simulink model "ControlsWithAutopilot_Properties"  (R2016a)
settings: Solver=ode45  StartTime=0.0  StopTime=10.0  RelTol=1e-3
undefined symbols (not defined in the file): ap, bias, DiscIntNeverNeededParam
libraries: simulink x3, discretizing x1
(part 1 of 3)
settings Model: Creator=mddavies  LastModifiedBy=Teme
settings DataIOCC: LimitDataPoints=on  SaveFormat=Array  SignalLoggingSaveFormat=ModelDataLogs
settings DebuggingCC: UnderspecifiedInitializationDetection=Classic  MergeDetectMultiDrivingBlocksExec=none  SolverPrmCheckMsg=warning  FcnCallInpInsideContextMsg=UseLocalSettings  StateNameClashWarn=warning
settings HardwareCC: ProdBitPerPointer=32  ProdLargestAtomicFloat=None  ProdIntDivRoundTo=Undefined  ProdEndianess=Unspecified  ProdWordSize=32  ProdHWDeviceType=32-bit Generic
settings ModelReferenceCC: PropagateSignalLabelsOutOfModel=off
settings GRTTargetCC: CombineOutputUpdateFcns=off  GRTInterface=on
settings ConfigComp: CovModelRefEnable=Off  CovSFcnEnable=off

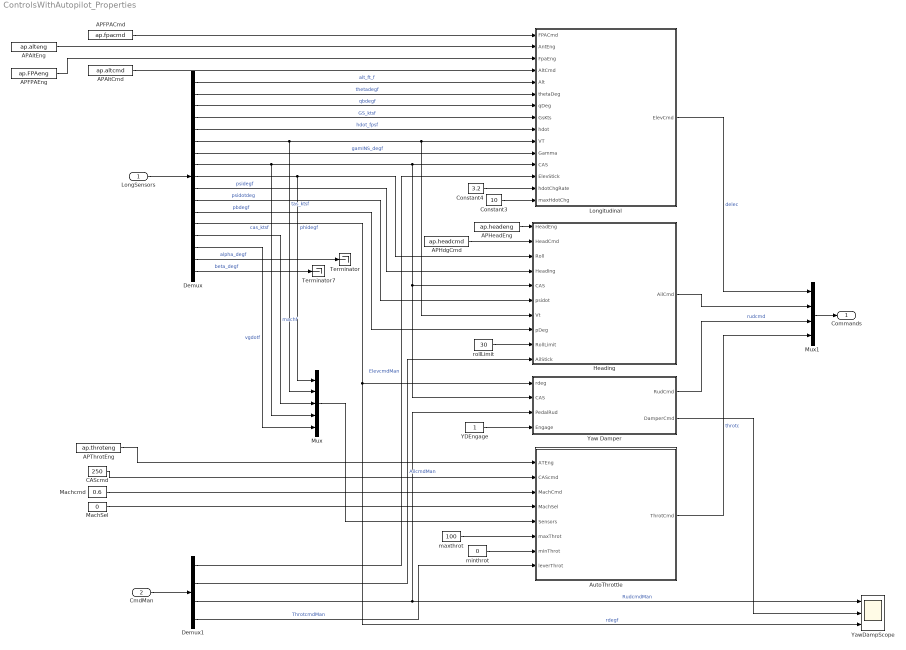
== system ControlsWithAutopilot_Properties ==
  LongSensors : Inport  RequirementInfo={} %GIDa_0ce9b168_5661_42b0_b4cb_7d3faaf2df72  PortDimensions=17
  CmdMan : Inport  RequirementInfo={} %GIDa_0ce9b168_5661_42b0_b4cb_7d3faaf2df72  Port=2  PortDimensions=9
  APAltCmd : Constant  RequirementInfo={} %GIDa_8396ea73_c2c1_410d_8e72_0a2c2e115229  Value=ap.altcmd
  APAltEng : Constant  RequirementInfo={} %GIDa_7acdc276_5904_4f5d_a4d8_b7eafc22dcba  Value=ap.alteng  OutDataTypeStr=boolean
  "APFPACmd " : Constant  RequirementInfo={} %GIDa_f2a9802e_c9ff_44b4_9c39_101c70e3085f  Value=ap.fpacmd
  APFPAEng : Constant  RequirementInfo={} %GIDa_b6347d6f_b14e_46b8_b79f_c4482e372009  Value=ap.FPAeng  OutDataTypeStr=boolean
  APHdgCmd : Constant  RequirementInfo={} %GIDa_ca348917_806b_4c73_b099_958ce531bbd5  Value=ap.headcmd
  APHeadEng : Constant  RequirementInfo={} %GIDa_019c8883_de5f_448b_a478_e0a40c975d97  Value=ap.headeng  OutDataTypeStr=boolean
  APThrotEng : Constant  RequirementInfo={} %GIDa_c34ca1b2_b760_48cb_8815_eaf096d766de  Value=ap.throteng  OutDataTypeStr=boolean
  AutoThrottle : Subsystem  RequirementInfo={'other' '..\..\tcm_requirements.docx' '@Simulink_requirement_item_20' 'true' 'Auto Throttle' '' } %GIDa_9e91f8aa_3697_4e86_a547_8b20eda6b794  TreatAsAtomicUnit=on
  CAScmd : Constant  RequirementInfo={} %GIDa_47d34f1f_8d24_42cb_857b_a6284aa9b10f  Value=250
  Constant3 : Constant  RequirementInfo={} %GIDa_6046f9e1_21da_4401_862c_288f604e8689  Value=10
  Constant4 : Constant  RequirementInfo={} %GIDa_dee93be0_a932_4ef0_a207_8f7329b01ca5  Value=3.2
  Demux : Demux  Outputs=17
  Demux1 : Demux
  Heading : Subsystem  TreatAsAtomicUnit=on
  Longitudinal : Subsystem  TreatAsAtomicUnit=on
  MachSel : Constant  RequirementInfo={} %GIDa_703eecf9_8ffd_4677_9df1_b11ad3ff81be  Value=0
  Machcmd : Constant  RequirementInfo={} %GIDa_a015b01e_abfd_4965_a258_bc3318cb77ef  Value=0.6
  Mux : Mux  Inputs=5
  Mux1 : Mux
  Terminator : Terminator
  Terminator7 : Terminator
      settings: RequirementInfo={} %GIDa_ea750fcf_3a35_4ca3_ba61_16c7ba83d83d
  YDEngage : Constant  RequirementInfo={} %GIDa_1b340559_9c71_403c_9901_bf0a93e2b9fd  SampleTime=-1
  Yaw Damper : Subsystem  RequirementInfo={'other' '..\..\tcm_requirements.docx' '@Simulink_requirement_item_19' 'true' 'Yaw Damper' '' } %GIDa_4d9fd165_a151_41ab_8542_450c342372eb  TreatAsAtomicUnit=on
  YawDampScope : Scope  NumInputPorts=3
      settings: RequirementInfo={} %GIDa_7592f6f2_c7e8_4acc_8768_b20cb3da46c8
  maxthrot : Constant  RequirementInfo={} %GIDa_230ab06c_3fb9_421e_bdda_8f032886ed67  Value=100  SampleTime=-1
  minthrot : Constant  RequirementInfo={} %GIDa_e24cf5cf_680d_403e_8bf4_a3705f2cf8ca  Value=0  SampleTime=-1
  rollLimit : Constant  RequirementInfo={} %GIDa_80188ac9_3eb7_4583_8db0_ebf7b7448de5  Value=30  SampleTime=-1
  Commands : Outport  RequirementInfo={} %GIDa_ba9bc9f0_2997_4cec_8a5a_2cb65716cddf
  wires:
  AutoThrottle/1(ThrotCmd) -> Mux1/4  "throtc"
  Longitudinal/1(ElevCmd) -> Mux1/1  "delec"
  Heading/1(AilCmd) -> Mux1/2
  CAScmd/1 -> AutoThrottle/2(CAScmd)
  APAltEng/1 -> Longitudinal/2(AntEng)
  Machcmd/1 -> AutoThrottle/3(MachCmd)
  MachSel/1 -> AutoThrottle/4(MachSel)
  APHeadEng/1 -> Heading/1(HeadEng)
  APFPAEng/1 -> Longitudinal/3(FpaEng)
  APThrotEng/1 -> AutoThrottle/1(ATEng)
  APHdgCmd/1 -> Heading/2(HeadCmd)
  "APFPACmd "/1 -> Longitudinal/1(FPACmd)
  APAltCmd/1 -> Longitudinal/4(AltCmd)
  maxthrot/1 -> AutoThrottle/6(maxThrot)
  Yaw Damper/2(DamperCmd) -> YawDampScope/2
  Yaw Damper/1(RudCmd) -> Mux1/3  "rudcmd"
  Constant3/1 -> Longitudinal/15(maxHdotChg)
  Constant4/1 -> Longitudinal/14(hdotChgRate)
  YDEngage/1 -> Yaw Damper/4(Engage)
  rollLimit/1 -> Heading/9(RollLimit)
  LongSensors/1 -> Demux/1
  Demux/1 -> Longitudinal/5(Alt)  "alt_ft_f"
  Demux/2 -> Longitudinal/6(thetaDeg)  "thetadegf"
  Demux/4 -> Longitudinal/8(GsKts)  "GS_ktsf"
  Demux/3 -> Longitudinal/7(qDeg)  "qbdegf"
  Demux/5 -> Longitudinal/9(hdot)  "hdot_fpsf"
  Demux/6 -> Longitudinal/10(VT), Heading/7(Vt), Mux/2  "tas_ktsf"
  Demux/7 -> Longitudinal/11(Gamma)  "gamINS_degf"
  Demux/8 -> Longitudinal/12(CAS), Yaw Damper/2(CAS), Heading/5(CAS), Mux/4  "cas_ktsf"
  Demux/16 -> Terminator/1  "alpha_degf"
  Demux/17 -> Terminator7/1  "beta_degf"
  Demux/9 -> Heading/3(Roll), Mux/1  "phidegf"
  Demux/10 -> Heading/4(Heading)  "psidegf"
  Demux/11 -> Heading/6(psidot)  "psidotdeg"
  Demux/12 -> Heading/8(pDeg)  "pbdegf"
  Demux/13 -> Yaw Damper/1(rdeg), YawDampScope/3  "rdegf"
  Demux/14 -> Mux/3  "machf"
  Demux/15 -> Mux/5  "vgdotf"
  minthrot/1 -> AutoThrottle/7(minThrot)
  CmdMan/1 -> Demux1/1
  Demux1/1 -> Longitudinal/13(ElevStick)  "ElevcmdMan"
  Demux1/2 -> Heading/10(AilStick)  "AilcmdMan"
  Demux1/3 -> YawDampScope/1, Yaw Damper/3(PedalRud)  "RudcmdMan"
  Demux1/4 -> AutoThrottle/8(leverThrot)  "ThrotcmdMan"
  Mux/1 -> AutoThrottle/5(Sensors)
  Mux1/1 -> Commands/1

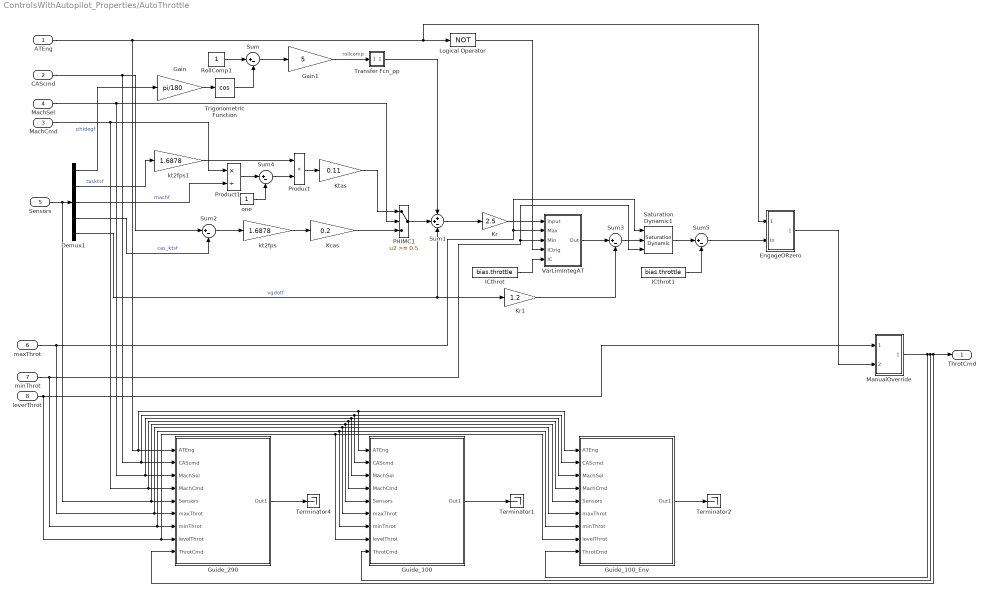
== system ControlsWithAutopilot_Properties/AutoThrottle ==
  ATEng : Inport  RequirementInfo={} %GIDa_2f45927d_6c28_4361_8173_5669474b9abd
  CAScmd : Inport  RequirementInfo={} %GIDa_92b5701d_5ed6_438c_8e94_843ad865eadf  Port=2
  MachCmd : Inport  RequirementInfo={} %GIDa_c26053c2_6b7f_4bf5_8f7d_768d0d646830  Port=3
  MachSel : Inport  RequirementInfo={} %GIDa_598b16f9_0dbe_4c96_859f_7e96536c1fb2  Port=4
  Sensors : Inport  RequirementInfo={} %GIDa_a55eff7f_fb2b_4f7a_a83b_479b402cff39  Port=5
  maxThrot : Inport  Port=6
  minThrot : Inport  Port=7
  leverThrot : Inport  Port=8
  Demux1 : Demux  Outputs=5
  EngageORzero : Subsystem
  Gain : Gain  RequirementInfo={} %GIDa_44ece66a_e9b1_47ae_9399_459633f82831  Gain=pi/180
  Gain1 : Gain  RequirementInfo={} %GIDa_5f70482a_3c80_415d_8392_528447a4813a  Gain=5
  Guide_100 : Subsystem  TreatAsAtomicUnit=on  mask(Observer){AnnotationType=ensures, ObserverType=ellipsoid}
      mask prompts: AnnotationType "Type of annotation (pre/post...)"; ObserverType "Observer type"
      mask help:
      | Set an observer for the system.
      | The annotation type parameter sets the type of observer:
      | - requires : pre-condition
      | - ensures : post-condition
      | - assert : an assertion
      | - observer : the observer computes a special type of properties
      mask TypeOptions AnnotationType: ensures | requires | assert | observer
      mask Callback AnnotationType:
      | paramStr = get_param(gcb, 'MaskValues');
      | 
      | if strcmp(paramStr{1}(1),'o')
      |     set_param(gcb,'MaskVisibilities',{'on';'on'});
      |     paramStr{2} = 'ellipsoid';
      |     set_param(gcb,'MaskValues',paramStr);
      | else
      |     set_param(gcb,'MaskVisibilities',{'on';'off'});
      | end
      mask Callback ObserverType:
      | paramStr = get_param(gcb, 'MaskValues');
      | 
      | if strcmp(paramStr{1}(1),'observer')
      |     set_param(gcb,'MaskVisibilities',{'on';'on'});
      |     paramStr{2} = 'ellipsoid';
      |     set_param(gcb,'MaskValues',paramStr);
      | else
      |     set_param(gcb,'MaskVisibilities',{'on';'off'});
      | end
      mask Display:
      | color('red');
      | text(0.5, 0.5, 'Observer Block', 'horizontalAlignment', 'center');
  Guide_100_Env : Subsystem  TreatAsAtomicUnit=on  mask(Observer){AnnotationType=ensures, ObserverType=ellipsoid}
      mask prompts: AnnotationType "Type of annotation (pre/post...)"; ObserverType "Observer type"
      mask help:
      | Set an observer for the system.
      | The annotation type parameter sets the type of observer:
      | - requires : pre-condition
      | - ensures : post-condition
      | - assert : an assertion
      | - observer : the observer computes a special type of properties
      mask TypeOptions AnnotationType: ensures | requires | assert | observer
      mask Callback AnnotationType:
      | paramStr = get_param(gcb, 'MaskValues');
      | 
      | if strcmp(paramStr{1}(1),'o')
      |     set_param(gcb,'MaskVisibilities',{'on';'on'});
      |     paramStr{2} = 'ellipsoid';
      |     set_param(gcb,'MaskValues',paramStr);
      | else
      |     set_param(gcb,'MaskVisibilities',{'on';'off'});
      | end
      mask Callback ObserverType:
      | paramStr = get_param(gcb, 'MaskValues');
      | 
      | if strcmp(paramStr{1}(1),'observer')
      |     set_param(gcb,'MaskVisibilities',{'on';'on'});
      |     paramStr{2} = 'ellipsoid';
      |     set_param(gcb,'MaskValues',paramStr);
      | else
      |     set_param(gcb,'MaskVisibilities',{'on';'off'});
      | end
      mask Display:
      | color('red');
      | text(0.5, 0.5, 'Observer Block', 'horizontalAlignment', 'center');
  Guide_290 : Subsystem  TreatAsAtomicUnit=on  mask(Observer){AnnotationType=ensures, ObserverType=ellipsoid}
      mask prompts: AnnotationType "Type of annotation (pre/post...)"; ObserverType "Observer type"
      mask help:
      | Set an observer for the system.
      | The annotation type parameter sets the type of observer:
      | - requires : pre-condition
      | - ensures : post-condition
      | - assert : an assertion
      | - observer : the observer computes a special type of properties
      mask TypeOptions AnnotationType: ensures | requires | assert | observer
      mask Callback AnnotationType:
      | paramStr = get_param(gcb, 'MaskValues');
      | 
      | if strcmp(paramStr{1}(1),'o')
      |     set_param(gcb,'MaskVisibilities',{'on';'on'});
      |     paramStr{2} = 'ellipsoid';
      |     set_param(gcb,'MaskValues',paramStr);
      | else
      |     set_param(gcb,'MaskVisibilities',{'on';'off'});
      | end
      mask Callback ObserverType:
      | paramStr = get_param(gcb, 'MaskValues');
      | 
      | if strcmp(paramStr{1}(1),'observer')
      |     set_param(gcb,'MaskVisibilities',{'on';'on'});
      |     paramStr{2} = 'ellipsoid';
      |     set_param(gcb,'MaskValues',paramStr);
      | else
      |     set_param(gcb,'MaskVisibilities',{'on';'off'});
      | end
      mask Display:
      | color('red');
      | text(0.5, 0.5, 'Observer Block', 'horizontalAlignment', 'center');
  ICthrot : Constant  RequirementInfo={} %GIDa_a96462ac_b28c_4fce_82e8_5e3952049bfb  Value=bias.throttle  SampleTime=-1
  ICthrot1 : Constant  RequirementInfo={} %GIDa_23dd534b_a590_436c_b15f_58e24838e8f2  Value=bias.throttle  SampleTime=-1
  Kcas : Gain  RequirementInfo={} %GIDa_1e6984b9_9479_49b0_970a_973f7c32edb7  Gain=0.2
  Kr : Gain  RequirementInfo={} %GIDa_18afb4c5_511e_47fb_85e5_bdfbcffb89de  Gain=2.5
  Kr1 : Gain  RequirementInfo={} %GIDa_9e9297b4_8c75_4533_a8dd_3891075538e5  Gain=1.2
  Ktas : Gain  RequirementInfo={} %GIDa_43c0fedf_b3e4_4e0f_a6fc_568c741b4ee2  Gain=0.11
  Logical Operator : Logic  RequirementInfo={} %GIDa_18e0a705_4fb5_4f14_a12b_8f6e047bc903  Operator=NOT  AllPortsSameDT=off  OutDataTypeStr=boolean
  ManualOverride : Subsystem
  PHIMC1 : Switch  RequirementInfo={} %GIDa_e2112eb0_c2db_4683_9846_bc0eb97a67f4  Threshold=0.5  SampleTime=0.02  SaturateOnIntegerOverflow=on
  Product : Product  RequirementInfo={} %GIDa_f2e51a99_89d7_4199_acd2_75b4a5a762fd  RndMeth=Zero
  Product1 : Product  RequirementInfo={} %GIDa_5c94e278_e588_4429_922d_3903b6601868  Inputs=*/  RndMeth=Zero
  RollComp1 : Constant  RequirementInfo={} %GIDa_8f810878_51f3_4d16_a407_aaec8ff4cd8a  SampleTime=-1
  Saturation Dynamic1 : simulink/Discontinuities/Saturation Dynamic  OutMin=[]  OutMax=[]  OutDataTypeStr=Inherit: Same as second input  OutDataType=sfix(16)  OutScaling=2^-10  DoSatur=off
  Sum : Sum  RequirementInfo={} %GIDa_9c88a12f_8eea_40db_a15a_aac24376aa7e  Inputs=|+-
  Sum1 : Sum  RequirementInfo={} %GIDa_fc0b036c_eb6d_4b0a_a40d_b7183183f1bc  Inputs=++-
  Sum2 : Sum  RequirementInfo={} %GIDa_95fcf8e7_99a7_46b3_9e41_77bfb2af0e6e  Inputs=|+-
  Sum3 : Sum  RequirementInfo={} %GIDa_0620e5c6_0d29_4c42_bdd5_2c680788712f  Inputs=|+-
  Sum4 : Sum  RequirementInfo={} %GIDa_a4cfd5ae_8cc7_4a4b_9229_0e28a225e0c7  Inputs=|+-
  Sum5 : Sum  RequirementInfo={} %GIDa_9cd0e9e4_7a0b_4a48_8c2a_57da4ad43678  Inputs=|+-
  Terminator1 : Terminator
  Terminator2 : Terminator
  Terminator4 : Terminator
  Transfer Fcn_pp : Subsystem  TreatAsAtomicUnit=on
  Trigonometric Function : Trigonometry  RequirementInfo={} %GIDa_82d3b8e2_fba4_4fde_a324_6f5a5fa38b0e  Operator=cos
  VarLimIntegAT : Subsystem  RequirementInfo={} %GIDa_946bbead_442f_495f_943e_e8a8eb5a05a2  TreatAsAtomicUnit=on
  kt2fps : Gain  RequirementInfo={} %GIDa_719dda5c_99e9_4155_8171_b1c9b5878f3a  Gain=1.6878
  kt2fps1 : Gain  RequirementInfo={} %GIDa_b06df2d8_ff63_4d20_83d9_1b3d18a391c7  Gain=1.6878
  one : Constant  RequirementInfo={} %GIDa_79530773_343c_40ed_88d6_a702a3c8b7d7  SampleTime=-1
  ThrotCmd : Outport  RequirementInfo={} %GIDa_10832092_f513_4063_bf4d_710db5c9192f
  wires:
  CAScmd/1 -> Sum2/1, Guide_290/2(CAScmd), Guide_100/2(CAScmd), Guide_100_Env/2(CAScmd)
  Sum2/1 -> kt2fps/1
  Sum1/1 -> Kr/1
  kt2fps/1 -> Kcas/1
  Kr/1 -> VarLimIntegAT/1(Input)
  Kr1/1 -> Sum3/2
  Gain1/1 -> Transfer Fcn_pp/1(Inport1)  "rollcomp"
  Sum/1 -> Gain1/1
  Trigonometric Function/1 -> Sum/2
  RollComp1/1 -> Sum/1
  Gain/1 -> Trigonometric Function/1
  Product1/1 -> Sum4/1
  one/1 -> Sum4/2
  Sum4/1 -> Product/2
  kt2fps1/1 -> Product/1
  Product/1 -> Ktas/1
  ICthrot/1 -> VarLimIntegAT/5(IC)
  Sum5/1 -> EngageORzero/2(In)
  ICthrot1/1 -> Sum5/2
  maxThrot/1 -> VarLimIntegAT/2(Max), Saturation Dynamic1/1, Guide_290/6(maxThrot), Guide_100/6(maxThrot), Guide_100_Env/6(maxThrot)
  minThrot/1 -> VarLimIntegAT/3(Min), Saturation Dynamic1/3, Guide_290/7(minThrot), Guide_100/7(minThrot), Guide_100_Env/7(minThrot)
  VarLimIntegAT/1(Out) -> Sum3/1
  Sum3/1 -> Saturation Dynamic1/2
  Saturation Dynamic1/1 -> Sum5/1
  PHIMC1/1 -> Sum1/2
  Kcas/1 -> PHIMC1/3
  Ktas/1 -> PHIMC1/1
  Transfer Fcn_pp/1(Outport1) -> Sum1/1
  Logical Operator/1 -> VarLimIntegAT/4(ICtrig)
  ATEng/1 -> EngageORzero/1(Engage), Logical Operator/1, Guide_290/1(ATEng), Guide_100/1(ATEng), Guide_100_Env/1(ATEng)
  MachSel/1 -> PHIMC1/2, Guide_290/3(MachSel), Guide_100/3(MachSel), Guide_100_Env/3(MachSel)
  MachCmd/1 -> Product1/1, Guide_290/4(MachCmd), Guide_100/4(MachCmd), Guide_100_Env/4(MachCmd)
  leverThrot/1 -> ManualOverride/1(Man), Guide_290/8(levelThrot), Guide_100/8(levelThrot), Guide_100_Env/8(levelThrot)
  ManualOverride/1(Out) -> ThrotCmd/1, Guide_290/9(ThrotCmd), Guide_100/9(ThrotCmd), Guide_100_Env/9(ThrotCmd)
  EngageORzero/1(Out) -> ManualOverride/2(Auto)
  Sensors/1 -> Demux1/1, Guide_290/5(Sensors), Guide_100/5(Sensors), Guide_100_Env/5(Sensors)
  Demux1/1 -> Gain/1  "phidegf"
  Demux1/2 -> kt2fps1/1  "tasktsf"
  Demux1/3 -> Product1/2  "machf"
  Demux1/4 -> Sum2/2  "cas_ktsf"
  Demux1/5 -> Sum1/3, Kr1/1  "vgdotf"
  Guide_290/1(Out1) -> Terminator4/1
  Guide_100/1(Out1) -> Terminator1/1
  Guide_100_Env/1(Out1) -> Terminator2/1

== system ControlsWithAutopilot_Properties/Heading ==
  HeadEng : Inport
  HeadCmd : Inport  Port=2
  Roll : Inport  Port=3
  Heading : Inport  Port=4
  CAS : Inport  Port=5
  psidot : Inport  Port=6
  Vt : Inport  Port=7
  pDeg : Inport  Port=8
  RollLimit : Inport  Port=9
  AilStick : Inport  Port=10
  EngageORzero : Subsystem
  Gain1 : Gain  RequirementInfo={} %GIDa_2f421c02_996e_46c9_ac2a_3c25b016b229  Gain=-1  SaturateOnIntegerOverflow=on  OutDataTypeStr=Inherit: Same as input  ParamDataTypeStr=Inherit: Same as input
  Guide_110 : Subsystem  TreatAsAtomicUnit=on  mask(Observer){AnnotationType=ensures, ObserverType=ellipsoid}
      mask prompts: AnnotationType "Type of annotation (pre/post...)"; ObserverType "Observer type"
      mask help:
      | Set an observer for the system.
      | The annotation type parameter sets the type of observer:
      | - requires : pre-condition
      | - ensures : post-condition
      | - assert : an assertion
      | - observer : the observer computes a special type of properties
      mask TypeOptions AnnotationType: ensures | requires | assert | observer
      mask Callback AnnotationType:
      | paramStr = get_param(gcb, 'MaskValues');
      | 
      | if strcmp(paramStr{1}(1),'o')
      |     set_param(gcb,'MaskVisibilities',{'on';'on'});
      |     paramStr{2} = 'ellipsoid';
      |     set_param(gcb,'MaskValues',paramStr);
      | else
      |     set_param(gcb,'MaskVisibilities',{'on';'off'});
      | end
      mask Callback ObserverType:
      | paramStr = get_param(gcb, 'MaskValues');
      | 
      | if strcmp(paramStr{1}(1),'observer')
      |     set_param(gcb,'MaskVisibilities',{'on';'on'});
      |     paramStr{2} = 'ellipsoid';
      |     set_param(gcb,'MaskValues',paramStr);
      | else
      |     set_param(gcb,'MaskVisibilities',{'on';'off'});
      | end
      mask Display:
      | color('red');
      | text(0.5, 0.5, 'Observer Block', 'horizontalAlignment', 'center');
  Heading Control : Subsystem  RequirementInfo={'other' '..\..\tcm_requirements.docx' '@Simulink_requirement_item_16' 'true' 'Heading Control' '' } %GIDa_911b8f78_7600_4481_9e93_a11b2a64dbe5  TreatAsAtomicUnit=on
  ManualOverride : Subsystem
  Roll InnerLoop : Subsystem  RequirementInfo={'other' '..\..\tcm_requirements.docx' '@Simulink_requirement_item_18' 'true' 'Roll InnerLoop' '' } %GIDa_311280c1_10c2_4ab3_a776_5e785b9037f8  TreatAsAtomicUnit=on
  Terminator2 : Terminator
  AilCmd : Outport
  wires:
  pDeg/1 -> Roll InnerLoop/3(pdeg), Guide_110/1(pbdegf)
  Vt/1 -> Heading Control/4(Vt), Guide_110/9(Vt)
  psidot/1 -> Heading Control/3(psidot), Guide_110/8(psidot)
  Heading/1 -> Heading Control/2(Heading), Guide_110/7(Heading)
  Roll/1 -> Heading Control/5(Roll), Roll InnerLoop/2(Roll), Guide_110/4(phidegf)
  Heading Control/1(RollCmd) -> Roll InnerLoop/1(RollCmd)
  Roll InnerLoop/1(AilCmd) -> EngageORzero/2(In)  "ailcmd"
  HeadEng/1 -> EngageORzero/1(Engage), Heading Control/6(HeadEng), Guide_110/5(HeadEng)
  CAS/1 -> Roll InnerLoop/4(CAS), Guide_110/2(CAS)
  RollLimit/1 -> Heading Control/7(RollLimit), Guide_110/3(RollLimit)
  ManualOverride/1(Out) -> Gain1/1
  AilStick/1 -> ManualOverride/1(Man), Guide_110/10(AilStick)
  Gain1/1 -> AilCmd/1, Guide_110/11(AilCmd)
  EngageORzero/1(Out) -> ManualOverride/2(Auto)
  HeadCmd/1 -> Heading Control/1(HdgCmdMCP), Guide_110/6(HeadCmd)
  Guide_110/1(Guide_110) -> Terminator2/1

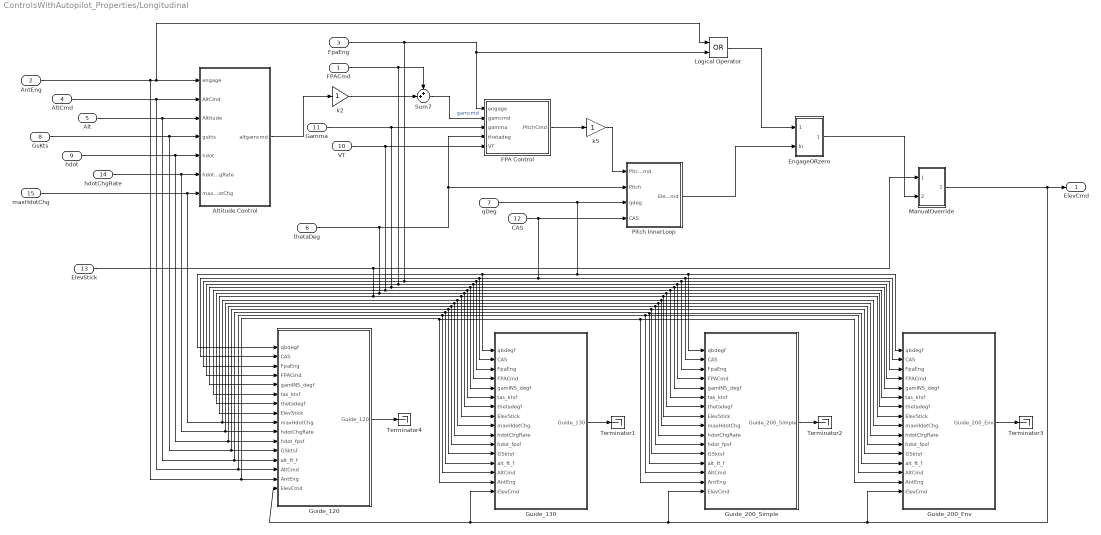
== system ControlsWithAutopilot_Properties/Longitudinal ==
  FPACmd : Inport
  AntEng : Inport  Port=2
  FpaEng : Inport  Port=3
  AltCmd : Inport  Port=4
  Alt : Inport  Port=5
  thetaDeg : Inport  Port=6
  qDeg : Inport  Port=7
  GsKts : Inport  Port=8
  hdot : Inport  Port=9
  VT : Inport  Port=10
  Gamma : Inport  Port=11
  CAS : Inport  Port=12
  ElevStick : Inport  Port=13
  hdotChgRate : Inport  Port=14
  maxHdotChg : Inport  Port=15
  Altitude Control : Subsystem  RequirementInfo={'other' '..\..\tcm_requirements.docx' '@Simulink_requirement_item_14' 'true' 'Altitude Control' '' } %GIDa_440f81f7_8b55_4c78_bea7_52c909831264  TreatAsAtomicUnit=on
  EngageORzero : Subsystem
  FPA Control : Subsystem  RequirementInfo={'other' '..\..\tcm_requirements.docx' '@Simulink_requirement_item_15' 'true' 'FPA Control' '' } %GIDa_71e3e321_cc66_4d8a_a4f3_fd2e7f1fbaff  TreatAsAtomicUnit=on
  Guide_120 : Subsystem  TreatAsAtomicUnit=on  mask(Observer){AnnotationType=ensures, ObserverType=ellipsoid}
      mask prompts: AnnotationType "Type of annotation (pre/post...)"; ObserverType "Observer type"
      mask help:
      | Set an observer for the system.
      | The annotation type parameter sets the type of observer:
      | - requires : pre-condition
      | - ensures : post-condition
      | - assert : an assertion
      | - observer : the observer computes a special type of properties
      mask TypeOptions AnnotationType: ensures | requires | assert | observer
      mask Callback AnnotationType:
      | paramStr = get_param(gcb, 'MaskValues');
      | 
      | if strcmp(paramStr{1}(1),'o')
      |     set_param(gcb,'MaskVisibilities',{'on';'on'});
      |     paramStr{2} = 'ellipsoid';
      |     set_param(gcb,'MaskValues',paramStr);
      | else
      |     set_param(gcb,'MaskVisibilities',{'on';'off'});
      | end
      mask Callback ObserverType:
      | paramStr = get_param(gcb, 'MaskValues');
      | 
      | if strcmp(paramStr{1}(1),'observer')
      |     set_param(gcb,'MaskVisibilities',{'on';'on'});
      |     paramStr{2} = 'ellipsoid';
      |     set_param(gcb,'MaskValues',paramStr);
      | else
      |     set_param(gcb,'MaskVisibilities',{'on';'off'});
      | end
      mask Display:
      | color('red');
      | text(0.5, 0.5, 'Observer Block', 'horizontalAlignment', 'center');
  Guide_130 : Subsystem  TreatAsAtomicUnit=on  mask(Observer){AnnotationType=ensures, ObserverType=ellipsoid}
      mask prompts: AnnotationType "Type of annotation (pre/post...)"; ObserverType "Observer type"
      mask help:
      | Set an observer for the system.
      | The annotation type parameter sets the type of observer:
      | - requires : pre-condition
      | - ensures : post-condition
      | - assert : an assertion
      | - observer : the observer computes a special type of properties
      mask TypeOptions AnnotationType: ensures | requires | assert | observer
      mask Callback AnnotationType:
      | paramStr = get_param(gcb, 'MaskValues');
      | 
      | if strcmp(paramStr{1}(1),'o')
      |     set_param(gcb,'MaskVisibilities',{'on';'on'});
      |     paramStr{2} = 'ellipsoid';
      |     set_param(gcb,'MaskValues',paramStr);
      | else
      |     set_param(gcb,'MaskVisibilities',{'on';'off'});
      | end
      mask Callback ObserverType:
      | paramStr = get_param(gcb, 'MaskValues');
      | 
      | if strcmp(paramStr{1}(1),'observer')
      |     set_param(gcb,'MaskVisibilities',{'on';'on'});
      |     paramStr{2} = 'ellipsoid';
      |     set_param(gcb,'MaskValues',paramStr);
      | else
      |     set_param(gcb,'MaskVisibilities',{'on';'off'});
      | end
      mask Display:
      | color('red');
      | text(0.5, 0.5, 'Observer Block', 'horizontalAlignment', 'center');
  Guide_200_Env : Subsystem  TreatAsAtomicUnit=on  mask(Observer){AnnotationType=ensures, ObserverType=ellipsoid}
      mask prompts: AnnotationType "Type of annotation (pre/post...)"; ObserverType "Observer type"
      mask help:
      | Set an observer for the system.
      | The annotation type parameter sets the type of observer:
      | - requires : pre-condition
      | - ensures : post-condition
      | - assert : an assertion
      | - observer : the observer computes a special type of properties
      mask TypeOptions AnnotationType: ensures | requires | assert | observer
      mask Callback AnnotationType:
      | paramStr = get_param(gcb, 'MaskValues');
      | 
      | if strcmp(paramStr{1}(1),'o')
      |     set_param(gcb,'MaskVisibilities',{'on';'on'});
      |     paramStr{2} = 'ellipsoid';
      |     set_param(gcb,'MaskValues',paramStr);
      | else
      |     set_param(gcb,'MaskVisibilities',{'on';'off'});
      | end
      mask Callback ObserverType:
      | paramStr = get_param(gcb, 'MaskValues');
      | 
      | if strcmp(paramStr{1}(1),'observer')
      |     set_param(gcb,'MaskVisibilities',{'on';'on'});
      |     paramStr{2} = 'ellipsoid';
      |     set_param(gcb,'MaskValues',paramStr);
      | else
      |     set_param(gcb,'MaskVisibilities',{'on';'off'});
      | end
      mask Display:
      | color('red');
      | text(0.5, 0.5, 'Observer Block', 'horizontalAlignment', 'center');
  Guide_200_Simple : Subsystem  TreatAsAtomicUnit=on  mask(Observer){AnnotationType=ensures, ObserverType=ellipsoid}
      mask prompts: AnnotationType "Type of annotation (pre/post...)"; ObserverType "Observer type"
      mask help:
      | Set an observer for the system.
      | The annotation type parameter sets the type of observer:
      | - requires : pre-condition
      | - ensures : post-condition
      | - assert : an assertion
      | - observer : the observer computes a special type of properties
      mask TypeOptions AnnotationType: ensures | requires | assert | observer
      mask Callback AnnotationType:
      | paramStr = get_param(gcb, 'MaskValues');
      | 
      | if strcmp(paramStr{1}(1),'o')
      |     set_param(gcb,'MaskVisibilities',{'on';'on'});
      |     paramStr{2} = 'ellipsoid';
      |     set_param(gcb,'MaskValues',paramStr);
      | else
      |     set_param(gcb,'MaskVisibilities',{'on';'off'});
      | end
      mask Callback ObserverType:
      | paramStr = get_param(gcb, 'MaskValues');
      | 
      | if strcmp(paramStr{1}(1),'observer')
      |     set_param(gcb,'MaskVisibilities',{'on';'on'});
      |     paramStr{2} = 'ellipsoid';
      |     set_param(gcb,'MaskValues',paramStr);
      | else
      |     set_param(gcb,'MaskVisibilities',{'on';'off'});
      | end
      mask Display:
      | color('red');
      | text(0.5, 0.5, 'Observer Block', 'horizontalAlignment', 'center');
  Logical Operator : Logic  Operator=OR  AllPortsSameDT=off  OutDataTypeStr=boolean
  ManualOverride : Subsystem
  Pitch InnerLoop : Subsystem  RequirementInfo={'other' '..\..\tcm_requirements.docx' '@Simulink_requirement_item_17' 'true' 'Pitch InnerLoop' '' } %GIDa_fc56dd5e_d6cd_42fe_934f_e4aed2c76eb1  TreatAsAtomicUnit=on
  Sum7 : Sum  RequirementInfo={} %GIDa_92495686_3877_4412_b19f_22e099e095ee  Inputs=++|
  Terminator{1..4} (4 alike) : Terminator
  k2 : Gain  RequirementInfo={} %GIDa_7e514706_5da4_4f1f_bf6c_0050dd9ce76d
  k5 : Gain  RequirementInfo={} %GIDa_b8b0ba7d_7fd3_4b03_b740_56530c3187c8
  ElevCmd : Outport
  wires:
  k2/1 -> Sum7/2
  Alt/1 -> Altitude Control/3(Altitude), Guide_120/13(alt_ft_f), Guide_200_Env/13(alt_ft_f), Guide_200_Simple/13(alt_ft_f), Guide_130/13(alt_ft_f)
  thetaDeg/1 -> FPA Control/4(thetadeg), Pitch InnerLoop/2(Pitch), Guide_120/7(thetadegf), Guide_200_Env/7(thetadegf), Guide_200_Simple/7(thetadegf), Guide_130/7(thetadegf)
  Gamma/1 -> FPA Control/3(gamma), Guide_120/5(gamINS_degf), Guide_200_Env/5(gamINS_degf), Guide_200_Simple/5(gamINS_degf), Guide_130/5(gamINS_degf)
  AltCmd/1 -> Altitude Control/2(AltCmd), Guide_120/14(AltCmd), Guide_200_Simple/14(AltCmd), Guide_200_Env/14(AltCmd), Guide_130/14(AltCmd)
  ManualOverride/1(Out) -> ElevCmd/1, Guide_200_Env/16(ElevCmd), Guide_200_Simple/16(ElevCmd), Guide_120/16(ElevCmd), Guide_130/16(ElevCmd)
  Altitude Control/1(altgamcmd) -> k2/1
  FPA Control/1(PitchCmd) -> k5/1
  hdot/1 -> Altitude Control/5(hdot), Guide_120/11(hdot_fpsf), Guide_200_Env/11(hdot_fpsf), Guide_200_Simple/11(hdot_fpsf), Guide_130/11(hdot_fpsf)
  Sum7/1 -> FPA Control/2(gamcmd)  "gamcmd"
  qDeg/1 -> Pitch InnerLoop/3(qdeg), Guide_120/1(qbdegf), Guide_130/1(qbdegf), Guide_200_Env/1(qbdegf), Guide_200_Simple/1(qbdegf)
  GsKts/1 -> Altitude Control/4(gskts), Guide_120/12(GSktsf), Guide_200_Env/12(GSktsf), Guide_200_Simple/12(GSktsf), Guide_130/12(GSktsf)
  VT/1 -> FPA Control/5(VT), Guide_120/6(tas_ktsf), Guide_130/6(tas_ktsf), Guide_200_Env/6(tas_ktsf), Guide_200_Simple/6(tas_ktsf)
  FPACmd/1 -> Sum7/1, Guide_120/4(FPACmd), Guide_200_Env/4(FPACmd), Guide_200_Simple/4(FPACmd), Guide_130/4(FPACmd)
  k5/1 -> Pitch InnerLoop/1(PitchCmd)
  FpaEng/1 -> Logical Operator/2, FPA Control/1(engage), Guide_120/3(FpaEng), Guide_130/3(FpaEng), Guide_200_Env/3(FpaEng), Guide_200_Simple/3(FpaEng)
  CAS/1 -> Pitch InnerLoop/4(CAS), Guide_120/2(CAS), Guide_130/2(CAS), Guide_200_Env/2(CAS), Guide_200_Simple/2(CAS)
  AntEng/1 -> Logical Operator/1, Altitude Control/1(engage), Guide_120/15(AntEng), Guide_200_Env/15(AntEng), Guide_200_Simple/15(AntEng), Guide_130/15(AntEng)
  ElevStick/1 -> ManualOverride/1(Man), Guide_120/8(ElevStick), Guide_200_Env/8(ElevStick), Guide_200_Simple/8(ElevStick), Guide_130/8(ElevStick)
  Pitch InnerLoop/1(ElevCmd) -> EngageORzero/2(In)
  EngageORzero/1(Out) -> ManualOverride/2(Auto)
  Logical Operator/1 -> EngageORzero/1(Engage)
  maxHdotChg/1 -> Altitude Control/7(maxHdotChg), Guide_120/9(maxHdotChg), Guide_200_Env/9(maxHdotChg), Guide_200_Simple/9(maxHdotChg), Guide_130/9(maxHdotChg)
  hdotChgRate/1 -> Altitude Control/6(hdotChgRate), Guide_120/10(hdotChgRate), Guide_200_Env/10(hdotChgRate), Guide_200_Simple/10(hdotChgRate), Guide_130/10(hdotChgRate)
  Guide_120/1(Guide_120) -> Terminator4/1
  Guide_130/1(Guide_130) -> Terminator1/1
  Guide_200_Env/1(Guide_200_Env) -> Terminator3/1
  Guide_200_Simple/1(Guide_200_Simple) -> Terminator2/1

== system ControlsWithAutopilot_Properties/Yaw Damper ==
  rdeg : Inport  RequirementInfo={} %GIDa_aab456ca_baa8_40be_af7c_3007e2406789
  CAS : Inport  RequirementInfo={} %GIDa_ffc3df4d_90ed_429c_9905_ba1d5e1c6104  Port=2
  PedalRud : Inport  Port=3
  Engage : Inport  Port=4
  EngageORzero : Subsystem
  Kcas_pp : Subsystem  TreatAsAtomicUnit=on
  Kr : Gain  RequirementInfo={} %GIDa_e1600aee_198d_416e_b040_c3f06ae50aaa  Gain=1.25
  ManualOverride : Subsystem  TreatAsAtomicUnit=on
      settings: MinAlgLoopOccurrences=on
  Product : Product  RequirementInfo={} %GIDa_b93a6279_44c9_4030_b746_3332e584ca8b  RndMeth=Zero
  YD_wo_pp : Subsystem  TreatAsAtomicUnit=on
  RudCmd : Outport  RequirementInfo={} %GIDa_5d934514_ad75_43c8_8562_5e4d07d2a065
  DamperCmd : Outport  Port=2
  wires:
  rdeg/1 -> Kr/1
  CAS/1 -> Kcas_pp/1(In)
  Kcas_pp/1(Out) -> Product/2
  ManualOverride/1(Out) -> RudCmd/1
  Kr/1 -> YD_wo_pp/1(Inport1)
  YD_wo_pp/1(Outport1) -> Product/1
  EngageORzero/1(Out) -> ManualOverride/2(Auto), DamperCmd/1
  PedalRud/1 -> ManualOverride/1(Man)
  Engage/1 -> EngageORzero/1(Engage)
  Product/1 -> EngageORzero/2(In)

== system ControlsWithAutopilot_Properties/AutoThrottle/EngageORzero ==
  Engage : Inport
  In : Inport  Port=2
  Logical Operator5 : Logic  RequirementInfo={} %GIDa_13e72d9c_1630_4494_8181_04ea596767a9  AllPortsSameDT=off  OutDataTypeStr=boolean
  Switch1 : Switch  RequirementInfo={} %GIDa_d89bdcfc_1e33_494f_b3fe_e13e317b4b5d  Threshold=0.5
  zero10 : Constant  RequirementInfo={} %GIDa_d1e784f7_2146_48f6_874a_0add9f175ac2
  zero9 : Constant  RequirementInfo={} %GIDa_df8b3a8b_00d1_4891_87af_e83379ed0682  Value=0
  Out : Outport
  wires:
  Engage/1 -> Logical Operator5/1
  zero10/1 -> Logical Operator5/2
  zero9/1 -> Switch1/3
  In/1 -> Switch1/1
  Logical Operator5/1 -> Switch1/2
  Switch1/1 -> Out/1

== system ControlsWithAutopilot_Properties/AutoThrottle/Guide_100 ==
  ATEng : Inport
  CAScmd : Inport  Port=2
  MachSel : Inport  Port=3
  MachCmd : Inport  Port=4
  Sensors : Inport  Port=5
  maxThrot : Inport  Port=6
  minThrot : Inport  Port=7
  levelThrot : Inport  Port=8
  ThrotCmd : Inport  Port=9
  Constant : Constant  Value=0
  Logical Operator : Logic  Operator=OR  AllPortsSameDT=off  OutDataTypeStr=boolean
  Logical Operator2 : Logic  Operator=NOT  AllPortsSameDT=off  OutDataTypeStr=boolean
  Relational Operator : RelationalOperator  Operator=~=  OutDataTypeStr=boolean
  Terminator{,1..6} (7 alike) : Terminator
  Out1 : Outport
  wires:
  levelThrot/1 -> Terminator/1
  CAScmd/1 -> Terminator4/1
  MachSel/1 -> Terminator3/1
  MachCmd/1 -> Terminator2/1
  Sensors/1 -> Terminator1/1
  ATEng/1 -> Logical Operator2/1
  Logical Operator/1 -> Out1/1
  Logical Operator2/1 -> Logical Operator/1
  ThrotCmd/1 -> Relational Operator/1
  Constant/1 -> Relational Operator/2
  Relational Operator/1 -> Logical Operator/2
  minThrot/1 -> Terminator5/1
  maxThrot/1 -> Terminator6/1

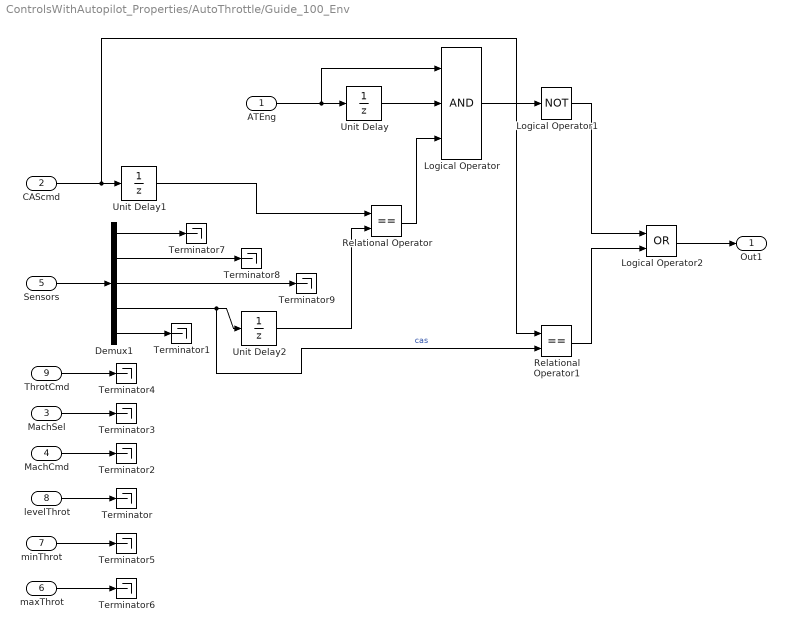
== system ControlsWithAutopilot_Properties/AutoThrottle/Guide_100_Env ==
  ATEng : Inport
  CAScmd : Inport  Port=2
  MachSel : Inport  Port=3
  MachCmd : Inport  Port=4
  Sensors : Inport  Port=5
  maxThrot : Inport  Port=6
  minThrot : Inport  Port=7
  levelThrot : Inport  Port=8
  ThrotCmd : Inport  Port=9
  Demux1 : Demux  Outputs=5
  Logical Operator : Logic  Inputs=3  AllPortsSameDT=off  OutDataTypeStr=boolean
  Logical Operator1 : Logic  Operator=NOT  AllPortsSameDT=off  OutDataTypeStr=boolean
  Logical Operator2 : Logic  Operator=OR  AllPortsSameDT=off  OutDataTypeStr=boolean
  Relational Operator : RelationalOperator  Operator===  OutDataTypeStr=boolean
  Relational Operator1 : RelationalOperator  Operator===  OutDataTypeStr=boolean
  Terminator{,1..9} (10 alike) : Terminator
  Unit Delay : UnitDelay
  Unit Delay1 : UnitDelay
  Unit Delay2 : UnitDelay
  Out1 : Outport
  wires:
  levelThrot/1 -> Terminator/1
  MachSel/1 -> Terminator3/1
  MachCmd/1 -> Terminator2/1
  Sensors/1 -> Demux1/1
  minThrot/1 -> Terminator5/1
  maxThrot/1 -> Terminator6/1
  Demux1/4 -> Unit Delay2/1, Relational Operator1/2  "cas"
  Demux1/3 -> Terminator9/1
  Demux1/2 -> Terminator8/1
  Demux1/1 -> Terminator7/1
  Demux1/5 -> Terminator1/1
  ATEng/1 -> Unit Delay/1, Logical Operator/1
  Unit Delay/1 -> Logical Operator/2
  CAScmd/1 -> Unit Delay1/1, Relational Operator1/1
  ThrotCmd/1 -> Terminator4/1
  Unit Delay1/1 -> Relational Operator/1
  Unit Delay2/1 -> Relational Operator/2
  Relational Operator/1 -> Logical Operator/3
  Logical Operator2/1 -> Out1/1
  Logical Operator1/1 -> Logical Operator2/1
  Logical Operator/1 -> Logical Operator1/1
  Relational Operator1/1 -> Logical Operator2/2

== system ControlsWithAutopilot_Properties/AutoThrottle/Guide_290 ==
  ATEng : Inport
  CAScmd : Inport  Port=2
  MachSel : Inport  Port=3
  MachCmd : Inport  Port=4
  Sensors : Inport  Port=5
  maxThrot : Inport  Port=6
  minThrot : Inport  Port=7
  levelThrot : Inport  Port=8
  ThrotCmd : Inport  Port=9
  Logical Operator : Logic  Operator=OR  AllPortsSameDT=off  OutDataTypeStr=boolean
  Logical Operator1 : Logic  AllPortsSameDT=off  OutDataTypeStr=boolean
  Logical Operator2 : Logic  Operator=NOT  AllPortsSameDT=off  OutDataTypeStr=boolean
  Relational Operator : RelationalOperator  Operator=<=  OutDataTypeStr=boolean
  Relational Operator1 : RelationalOperator  Operator=<=  OutDataTypeStr=boolean
  Terminator{,1..4} (5 alike) : Terminator
  Out1 : Outport
  wires:
  levelThrot/1 -> Terminator/1
  CAScmd/1 -> Terminator4/1
  MachSel/1 -> Terminator3/1
  MachCmd/1 -> Terminator2/1
  Sensors/1 -> Terminator1/1
  ATEng/1 -> Logical Operator2/1
  Logical Operator/1 -> Out1/1
  Logical Operator2/1 -> Logical Operator/1
  minThrot/1 -> Relational Operator/1
  ThrotCmd/1 -> Relational Operator/2, Relational Operator1/1
  maxThrot/1 -> Relational Operator1/2
  Relational Operator/1 -> Logical Operator1/1
  Relational Operator1/1 -> Logical Operator1/2
  Logical Operator1/1 -> Logical Operator/2

== system ControlsWithAutopilot_Properties/AutoThrottle/ManualOverride ==
  Man : Inport
  Auto : Inport  Port=2
  Switch1 : Switch  RequirementInfo={} %GIDa_99412258_89e8_4c84_a7a6_8adb3817b9de  Criteria=u2 ~= 0  Threshold=0.5
  Out : Outport
  wires:
  Man/1 -> Switch1/3, Switch1/2
  Auto/1 -> Switch1/1
  Switch1/1 -> Out/1

== system ControlsWithAutopilot_Properties/AutoThrottle/Transfer Fcn_pp ==
  Inport1 : Inport
  D1 : UnitDelay  SampleTime=-1
  GainAC1_1 : Gain  Gain=-0.0625  SaturateOnIntegerOverflow=on  OutDataTypeStr=Inherit: Same as input  ParamDataTypeStr=Inherit: Same as input
  GainAC2_1 : Gain  Gain=-0.0625  SaturateOnIntegerOverflow=on  OutDataTypeStr=Inherit: Same as input  ParamDataTypeStr=Inherit: Same as input
  GainBD1_1 : Gain  SaturateOnIntegerOverflow=on  OutDataTypeStr=Inherit: Same as input  ParamDataTypeStr=Inherit: Same as input
  GainBD2_1 : Gain  SaturateOnIntegerOverflow=on  OutDataTypeStr=Inherit: Same as input  ParamDataTypeStr=Inherit: Same as input
  Sum1 : Sum  SaturateOnIntegerOverflow=on  InputSameDT=on  OutDataTypeStr=Inherit: Same as first input
  Sum2 : Sum  SaturateOnIntegerOverflow=on  InputSameDT=on  OutDataTypeStr=Inherit: Same as first input
  Outport1 : Outport
  wires:
  D1/1 -> GainAC1_1/1, GainAC2_1/1
  GainAC1_1/1 -> Sum1/1
  GainAC2_1/1 -> Sum2/1
  Inport1/1 -> GainBD1_1/1, GainBD2_1/1
  GainBD1_1/1 -> Sum1/2
  GainBD2_1/1 -> Sum2/2
  Sum1/1 -> D1/1
  Sum2/1 -> Outport1/1

== system ControlsWithAutopilot_Properties/AutoThrottle/VarLimIntegAT ==
  Input : Inport  RequirementInfo={} %GIDa_91b38f96_ed38_45a6_8bb9_ff3fb81525df
  Max : Inport  RequirementInfo={} %GIDa_5200ce52_bb44_458c_9945_e382c2e773b4  Port=2
  Min : Inport  RequirementInfo={} %GIDa_600874e9_d5fd_4de5_b948_9284e9d56639  Port=3
  ICtrig : Inport  RequirementInfo={} %GIDa_af678c0a_424b_44b8_aa3a_3f303d846e8e  Port=4
  IC : Inport  RequirementInfo={} %GIDa_872b1a96_8436_4d34_8580_74ad3366301d  Port=5
  Constant1 : Constant  RequirementInfo={} %GIDa_bf704cc0_6bc9_4624_9fa4_e77befe43ee9  Value=0  SampleTime=-1
  Constant2 : Constant  RequirementInfo={} %GIDa_7032ed75_2ad3_41e5_9584_0891c369141c  Value=0  SampleTime=-1
  Constant3 : Constant  RequirementInfo={} %GIDa_f4367f96_4d82_41b7_8e43_0c6cec23a023  Value=0  SampleTime=-1
  Integrator1 : DiscreteIntegrator  ExternalReset=level  InitialConditionSource=external  SampleTime=1.0  ICPrevOutput=DiscIntNeverNeededParam  ICPrevScaledInput=DiscIntNeverNeededParam  mask(DiscretizedDiscreteIntegrator){}
      mask init:
      | %zoh
  Logical Operator1 : Logic  RequirementInfo={} %GIDa_53e2ecf2_1671_4b86_a4e6_7e9f03594f4a  Operator=OR
  Logical Operator2 : Logic  RequirementInfo={} %GIDa_f9639a17_73a7_4a19_b9c3_2b3e1bcf1152
  Logical Operator3 : Logic  RequirementInfo={} %GIDa_53705a9e_f0e6_4df8_b74a_51dda5b71ea0
  Relational Operator1 : RelationalOperator  RequirementInfo={} %GIDa_85cee0a0_d47b_41e2_b8dd_f48b296f5cf4  Operator=<=  InputSameDT=on
  Relational Operator2 : RelationalOperator  RequirementInfo={} %GIDa_74942223_cbc1_42b5_8e5e_e6b9112f9130  InputSameDT=on
  Relational Operator3 : RelationalOperator  RequirementInfo={} %GIDa_ea1202bb_7a42_4314_84fa_c36aa79c966a  Operator=>  InputSameDT=on
  Relational Operator4 : RelationalOperator  RequirementInfo={} %GIDa_c9e3adfb_bd3d_4cfe_9bd6_4a3fd1707fe2  Operator=<  InputSameDT=on
  Switch1 : Switch  RequirementInfo={} %GIDa_ed603307_5c4b_4569_8f05_95ce39b1df88  Threshold=0.1  SaturateOnIntegerOverflow=on  InputSameDT=on
  Out : Outport  RequirementInfo={} %GIDa_a7cb998d_eb28_45ce_8ac9_f1554f32fe4e
  wires:
  IC/1 -> Integrator1/3
  ICtrig/1 -> Integrator1/2
  Min/1 -> Relational Operator1/2
  Max/1 -> Relational Operator2/2
  Constant3/1 -> Relational Operator4/2
  Input/1 -> Switch1/3, Relational Operator3/1, Relational Operator4/1
  Logical Operator3/1 -> Logical Operator1/2
  Relational Operator4/1 -> Logical Operator3/2
  Relational Operator1/1 -> Logical Operator3/1
  Constant2/1 -> Relational Operator3/2
  Logical Operator2/1 -> Logical Operator1/1
  Relational Operator3/1 -> Logical Operator2/2
  Relational Operator2/1 -> Logical Operator2/1
  Logical Operator1/1 -> Switch1/2
  Integrator1/1 -> Relational Operator2/1, Relational Operator1/1, Out/1
  Switch1/1 -> Integrator1/1
  Constant1/1 -> Switch1/1

== system ControlsWithAutopilot_Properties/Heading/EngageORzero ==
  Engage : Inport
  In : Inport  Port=2
  Logical Operator5 : Logic  RequirementInfo={} %GIDa_7add67f6_200e_4459_8afc_a50a3802c341  AllPortsSameDT=off  OutDataTypeStr=boolean
  Switch1 : Switch  RequirementInfo={} %GIDa_a1777089_6daf_41d2_9e69_9356c4782e25  Threshold=0.5
  zero10 : Constant  RequirementInfo={} %GIDa_d889400f_b153_4cfc_a180_15b84145f1e0
  zero9 : Constant  RequirementInfo={} %GIDa_9027fd24_3b48_4acd_a774_517fb1aa3516  Value=0
  Out : Outport
  wires:
  Engage/1 -> Logical Operator5/1
  zero10/1 -> Logical Operator5/2
  zero9/1 -> Switch1/3
  In/1 -> Switch1/1
  Logical Operator5/1 -> Switch1/2
  Switch1/1 -> Out/1

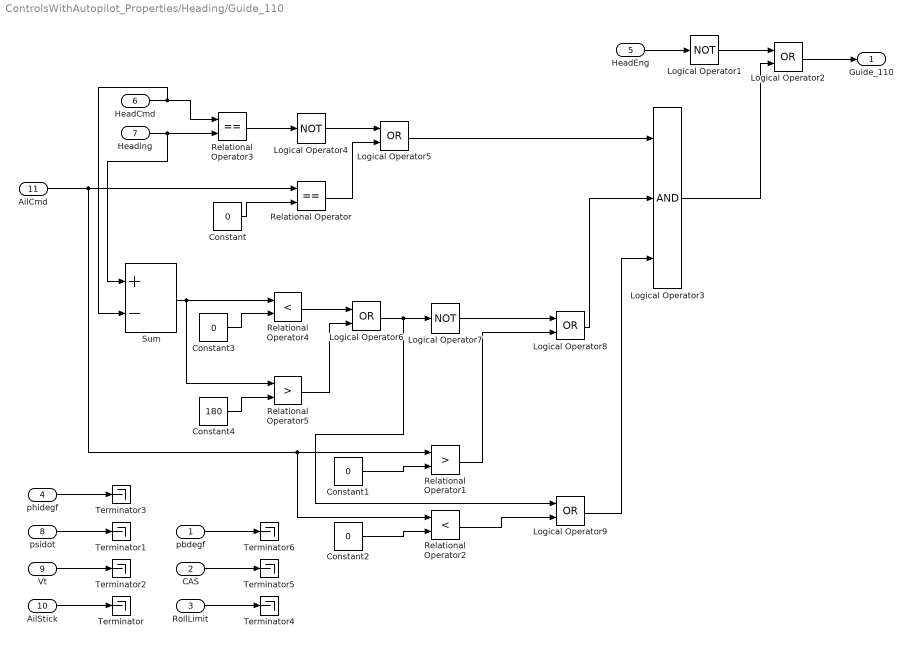
== system ControlsWithAutopilot_Properties/Heading/Guide_110 ==
  pbdegf : Inport
  CAS : Inport  Port=2
  RollLimit : Inport  Port=3
  phidegf : Inport  Port=4
  HeadEng : Inport  Port=5
  HeadCmd : Inport  Port=6
  Heading : Inport  Port=7
  psidot : Inport  Port=8
  Vt : Inport  Port=9
  AilStick : Inport  Port=10
  AilCmd : Inport  Port=11
  Constant{,1..3} (4 alike) : Constant  Value=0
  Constant4 : Constant  Value=180
  Logical Operator1 : Logic  Operator=NOT  AllPortsSameDT=off  OutDataTypeStr=boolean
  Logical Operator{2,5..6,8..9} (5 alike) : Logic  Operator=OR  AllPortsSameDT=off  OutDataTypeStr=boolean
  Logical Operator3 : Logic  Inputs=3  AllPortsSameDT=off  OutDataTypeStr=boolean
  Logical Operator4 : Logic  Operator=NOT  AllPortsSameDT=off  OutDataTypeStr=boolean
  Logical Operator7 : Logic  Operator=NOT  AllPortsSameDT=off  OutDataTypeStr=boolean
  Relational Operator : RelationalOperator  Operator===  OutDataTypeStr=boolean
  Relational Operator1 : RelationalOperator  Operator=>  OutDataTypeStr=boolean
  Relational Operator2 : RelationalOperator  Operator=<  OutDataTypeStr=boolean
  Relational Operator3 : RelationalOperator  Operator===  OutDataTypeStr=boolean
  Relational Operator4 : RelationalOperator  Operator=<  OutDataTypeStr=boolean
  Relational Operator5 : RelationalOperator  Operator=>  OutDataTypeStr=boolean
  Sum : Sum  Inputs=+-
  Terminator{,1..6} (7 alike) : Terminator
  Guide_110 : Outport
  wires:
  AilStick/1 -> Terminator/1
  Vt/1 -> Terminator2/1
  psidot/1 -> Terminator1/1
  phidegf/1 -> Terminator3/1
  RollLimit/1 -> Terminator4/1
  CAS/1 -> Terminator5/1
  pbdegf/1 -> Terminator6/1
  HeadEng/1 -> Logical Operator1/1
  Logical Operator1/1 -> Logical Operator2/1
  Logical Operator2/1 -> Guide_110/1
  AilCmd/1 -> Relational Operator/1, Relational Operator1/1, Relational Operator2/1
  Constant/1 -> Relational Operator/2
  Constant1/1 -> Relational Operator1/2
  Constant2/1 -> Relational Operator2/2
  Logical Operator4/1 -> Logical Operator5/1
  Relational Operator3/1 -> Logical Operator4/1
  Relational Operator/1 -> Logical Operator5/2
  Logical Operator5/1 -> Logical Operator3/1
  Sum/1 -> Relational Operator4/1, Relational Operator5/1
  Constant3/1 -> Relational Operator4/2
  Relational Operator4/1 -> Logical Operator6/1
  Constant4/1 -> Relational Operator5/2
  Relational Operator5/1 -> Logical Operator6/2
  HeadCmd/1 -> Relational Operator3/1, Sum/2
  Heading/1 -> Relational Operator3/2, Sum/1
  Logical Operator6/1 -> Logical Operator7/1, Logical Operator9/1
  Logical Operator7/1 -> Logical Operator8/1
  Relational Operator1/1 -> Logical Operator8/2
  Logical Operator8/1 -> Logical Operator3/2
  Relational Operator2/1 -> Logical Operator9/2
  Logical Operator9/1 -> Logical Operator3/3
  Logical Operator3/1 -> Logical Operator2/2
